simulink model "TRR_LQR"  (R2021a)
settings: Solver=FixedStepAuto  StartTime=0.0  StopTime=100000  FixedStep=.005  RelTol=1e-3  EnableMultiTasking=on
model workspace (MAT data in the model file):
  SL_ROS_VariableLengthArrays_MaxSizes.CommonInfo.ArrayTruncateAction = 'EmitWarning'
  SL_ROS_VariableLengthArrays_MaxSizes.MsgTypeMap = containers.Map
  SL_ROS_VariableLengthArrays_MaxSizes.MsgTypeMap.serialization.keys = {'sensor_msgs/JointState'}
  SL_ROS_VariableLengthArrays_MaxSizes.MsgTypeMap.serialization.values{1}(1).PropertyName = 'Effort'
  SL_ROS_VariableLengthArrays_MaxSizes.MsgTypeMap.serialization.values{1}(1).DataType = 'double'
  SL_ROS_VariableLengthArrays_MaxSizes.MsgTypeMap.serialization.values{1}(1).MaxLength = 128
  SL_ROS_VariableLengthArrays_MaxSizes.MsgTypeMap.serialization.values{1}(2).PropertyName = 'Name'
  SL_ROS_VariableLengthArrays_MaxSizes.MsgTypeMap.serialization.values{1}(2).DataType = 'std_msgs/String'
  SL_ROS_VariableLengthArrays_MaxSizes.MsgTypeMap.serialization.values{1}(2).MaxLength = 16
  SL_ROS_VariableLengthArrays_MaxSizes.MsgTypeMap.serialization.values{1}(3).PropertyName = 'Position'
  SL_ROS_VariableLengthArrays_MaxSizes.MsgTypeMap.serialization.values{1}(3).DataType = 'double'
  SL_ROS_VariableLengthArrays_MaxSizes.MsgTypeMap.serialization.values{1}(3).MaxLength = 3
  SL_ROS_VariableLengthArrays_MaxSizes.MsgTypeMap.serialization.values{1}(4).PropertyName = 'Velocity'
  SL_ROS_VariableLengthArrays_MaxSizes.MsgTypeMap.serialization.values{1}(4).DataType = 'double'
  SL_ROS_VariableLengthArrays_MaxSizes.MsgTypeMap.serialization.values{1}(4).MaxLength = 3
  SL_ROS_VariableLengthArrays_MaxSizes.MsgTypeMap.serialization.uniformity = 0
  SL_ROS_VariableLengthArrays_MaxSizes.MsgTypeMap.serialization.keyType = 'char'
  SL_ROS_VariableLengthArrays_MaxSizes.MsgTypeMap.serialization.valueType = 'any'
undefined symbols (not defined in the file): K
libraries: robotlib x7
settings Model: PacingRate=0.890000  Creator=Dr.Saraf  LastModifiedBy=reaperj
settings SolverCC: AlgebraicLoopSolver=TrustRegion
settings OptimizationCC: EnhancedBackFolding=on  PassReuseOutputArgsAs=Individual arguments  ZeroExternalMemoryAtStartup=off  ZeroInternalMemoryAtStartup=off  MaxStackSize=64  OptimizeBlockOrder=speed  DifferentSizesBufferReuse=on  OptimizationCustomize=off  EfficientTunableParamExpr=on
settings DebuggingCC: ParameterTunabilityLossMsg=error  SFMachineParentedDataDiag=warning
settings HardwareCC: ProdBitPerPointer=32  ProdBitPerSizeT=32  ProdBitPerPtrDiffT=32  ProdLargestAtomicFloat=None  ProdIntDivRoundTo=Undefined  ProdEndianess=Unspecified  ProdWordSize=32  ProdHWDeviceType=Generic->Unspecified (assume 32-bit Generic)  UseEmbeddedCoderFeatures=off
settings SFSimCC: MATLABDynamicMemAlloc=off
settings RTWCC: SystemTargetFile=ert.tlc  HardwareBoard=Robot Operating System (ROS)  TLCOptions="-aInlineSetEventsForThisBaseRateFcn=TLC_FALSE -aSuppressMultiTaskScheduler=TLC_FALSE  -aRateBasedStepFcn=0"  TemplateMakefile=ert_default_tmf  Toolchain=Catkin  TargetLang=C++
settings CodeAppCC: ForceParamTrailComments=on  IgnoreCustomStorageClasses=off  OperatorAnnotations=on  SimulinkDataObjDesc=on  SFDataObjDesc=on  InsertBlockDesc=on
settings ERTTargetCC: SupportNonInlinedSFcns=on

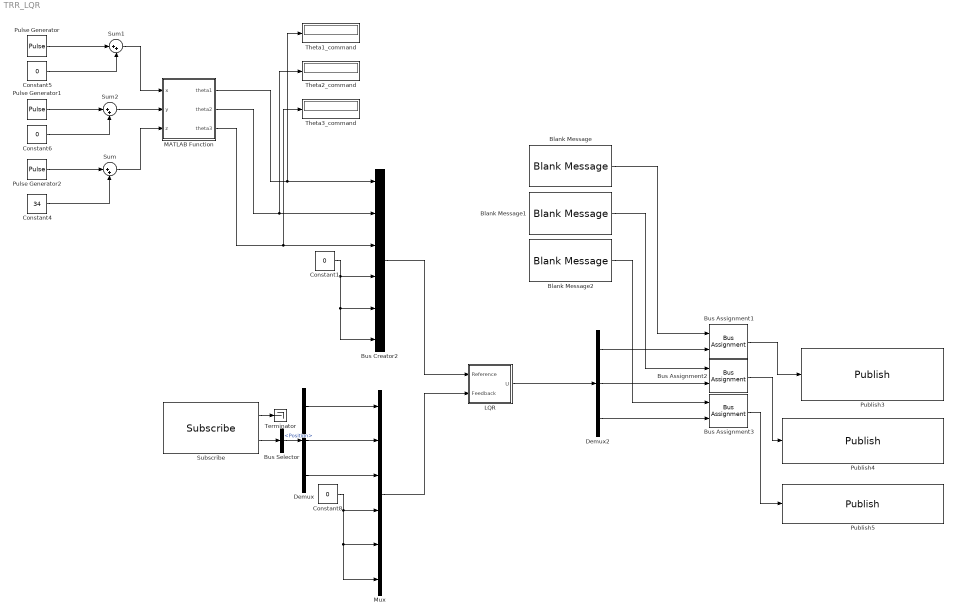
== system TRR_LQR ==
  Blank Message : robotlib/Blank Message  messageClass=Message  entityType=std_msgs/Float64  messageType=std_msgs/Float64  SampleTime=-1  legacyBusStruct=off
  Blank Message1 : robotlib/Blank Message  messageClass=Message  entityType=std_msgs/Float64  messageType=std_msgs/Float64  SampleTime=-1  legacyBusStruct=off
  Blank Message2 : robotlib/Blank Message  messageClass=Message  entityType=std_msgs/Float64  messageType=std_msgs/Float64  SampleTime=-1  legacyBusStruct=off
  Bus Assignment1 : BusAssignment  AssignedSignals=Data
  Bus Assignment2 : BusAssignment  AssignedSignals=Data
  Bus Assignment3 : BusAssignment  AssignedSignals=Data
  Bus Creator2 : BusCreator  Inputs=6
  Bus Selector : BusSelector  OutputSignals=Position
  Constant{1,5..6,8} (4 alike) : Constant  Value=0
  Constant4 : Constant  Value=34
  Demux : Demux  Outputs=3
  Demux2 : Demux  Outputs=3
  LQR : Subsystem
  MATLAB Function : MATLAB Function  TreatAsAtomicUnit=on
  Mux : Mux  Inputs=6
  Publish3 : robotlib/Publish  topicSource=Select from ROS network  topic=/iiwa/joint1_effort_controller/command  messageType=std_msgs/Float64  legacyBusStruct=off  messageQueueLength=3
  Publish4 : robotlib/Publish  topicSource=Select from ROS network  topic=/iiwa/joint2_effort_controller/command  messageType=std_msgs/Float64  legacyBusStruct=off  messageQueueLength=3
  Publish5 : robotlib/Publish  topicSource=Select from ROS network  topic=/iiwa/joint4_effort_controller/command  messageType=std_msgs/Float64  legacyBusStruct=off  messageQueueLength=3
  Pulse Generator : DiscretePulseGenerator  PulseType=Time based  Amplitude=-50  Period=10  PulseWidth=50
  Pulse Generator1 : DiscretePulseGenerator  PulseType=Time based  Amplitude=-50  Period=10  PulseWidth=50  PhaseDelay=5
  Pulse Generator2 : DiscretePulseGenerator  PulseType=Time based  Amplitude=40  Period=10  PulseWidth=50  PhaseDelay=5
  Subscribe : robotlib/Subscribe  topicSource=Select from ROS network  topic=/iiwa/joint_states  messageType=sensor_msgs/JointState  SampleTime=-1  legacyBusStruct=off  messageQueueLength=1
  Sum : Sum  Inputs=|++
  Sum1 : Sum  Inputs=|++
  Sum2 : Sum  Inputs=|++
  Terminator : Terminator
  Theta1_command : Display
  Theta2_command : Display
  Theta3_command : Display
  wires:
  Bus Creator2/1 -> LQR/1(Reference)
  Bus Assignment3/1 -> Publish5/1
  Blank Message2/1 -> Bus Assignment3/1
  Blank Message/1 -> Bus Assignment1/1
  Blank Message1/1 -> Bus Assignment2/1
  Bus Assignment2/1 -> Publish4/1
  Bus Assignment1/1 -> Publish3/1
  Sum/1 -> MATLAB Function/3(z)
  Mux/1 -> LQR/2(Feedback)
  Subscribe/1 -> Terminator/1
  MATLAB Function/3(theta3) -> Bus Creator2/3, Theta3_command/1
  MATLAB Function/2(theta2) -> Bus Creator2/2, Theta2_command/1
  MATLAB Function/1(theta1) -> Bus Creator2/1, Theta1_command/1
  LQR/1(U) -> Demux2/1
  Sum1/1 -> MATLAB Function/1(x)
  Sum2/1 -> MATLAB Function/2(y)
  Demux2/2 -> Bus Assignment2/2
  Demux2/1 -> Bus Assignment1/2
  Demux2/3 -> Bus Assignment3/2
  Constant8/1 -> Mux/6, Mux/5, Mux/4
  Subscribe/2 -> Bus Selector/1
  Demux/1 -> Mux/1
  Demux/2 -> Mux/2
  Bus Selector/1 -> Demux/1  "<Position>"
  Demux/3 -> Mux/3
  Constant6/1 -> Sum2/2
  Pulse Generator/1 -> Sum1/1
  Constant5/1 -> Sum1/2
  Pulse Generator2/1 -> Sum/1
  Pulse Generator1/1 -> Sum2/1
  Constant4/1 -> Sum/2
  Constant1/1 -> Bus Creator2/4, Bus Creator2/6, Bus Creator2/5

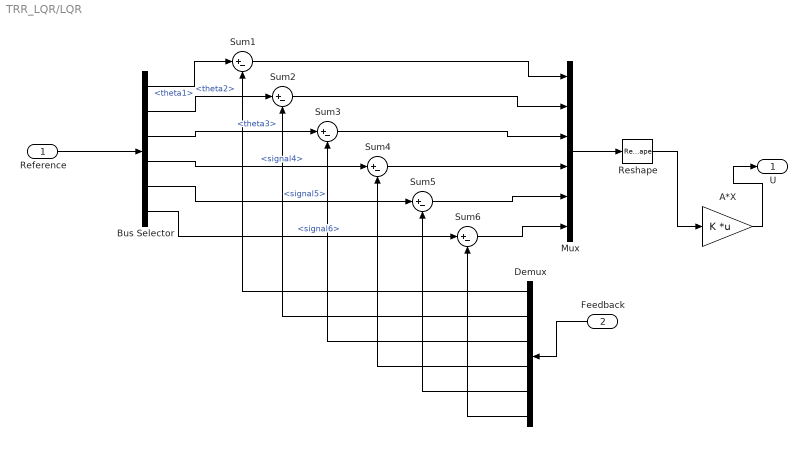
== system TRR_LQR/LQR ==
  Reference : Inport
  Feedback : Inport  Port=2
  A*X : Gain  Gain=K  Multiplication=Matrix(K*u)
  Bus Selector : BusSelector  OutputSignals=theta1,theta2,theta3,signal4,signal5,signal6
  Demux : Demux  Outputs=6
  Mux : Mux  Inputs=6
  Reshape : Reshape  OutputDimensionality=Column vector (2-D)
  Sum{1..6} (6 alike) : Sum  Inputs=|+-
  U : Outport
  wires:
  Sum2/1 -> Mux/2
  Sum6/1 -> Mux/6
  Sum3/1 -> Mux/3
  Sum5/1 -> Mux/5
  Sum4/1 -> Mux/4
  Bus Selector/6 -> Sum6/1  "<signal6>"
  Demux/5 -> Sum5/2
  Demux/3 -> Sum3/2
  Bus Selector/1 -> Sum1/1  "<theta1>"
  Sum1/1 -> Mux/1
  Demux/4 -> Sum4/2
  Demux/6 -> Sum6/2
  Bus Selector/2 -> Sum2/1  "<theta2>"
  Feedback/1 -> Demux/1
  Bus Selector/3 -> Sum3/1  "<theta3>"
  Bus Selector/5 -> Sum5/1  "<signal5>"
  Bus Selector/4 -> Sum4/1  "<signal4>"
  Reference/1 -> Bus Selector/1
  A*X/1 -> U/1
  Demux/1 -> Sum1/2
  Demux/2 -> Sum2/2
  Mux/1 -> Reshape/1
  Reshape/1 -> A*X/1

== matlab function TRR_LQR/MATLAB Function ==
  data: x input; theta1 output; y input; z input; theta2 output; theta3 output
%% Inverse Kinematics
function [theta1, theta2, theta3] = invk(x,y,z)

a1 = 34; a2 = 40; a3 = 52.6;

r1 = sqrt(x^2 + y^2);
r2 = a1 - z;
if(r1== 0 && r2>=0)
    phi2 = pi/2;
elseif(r1== 0 && r2<0)
    phi2 = -pi/2;
else
    phi2 = atan(r2/r1);
end

r3 = sqrt(r1^2 + r2^2);
if(r3== 0)
    phi1 = 0;
else
    phi1 = acos((a3^2 - a2^2 - r3^2)/(-2*a2*r3));
end

phi3 = acos((r3^2 - a2^2 - a3^2)/(-2*a2*a3));

if(y == 0)
    theta1 = 0 ;
else
    theta1 = atan(y/x);
end

theta2 = phi2 - phi1 ;
theta3 = - pi + phi3;

theta1 = theta1 + (pi/2) ;
theta2 = theta2 + (pi/2);


end
